simulink model "aaa"  (R2016b)
settings: Solver=ode4  StartTime=0.0  StopTime=inf  FixedStep=0.002  RelTol=1e-3  EnableMultiTasking=on
libraries: slrtlib x3
(part 5 of 5)

== stateflow chart aaa/tiaoshimoshi/jinjichuli7 ==
  state MANUAL
    state kaigai [parallel]
      settings: executionOrder=1
      state A
        entry:kghx=0;
      state on
        entry:kghx=1;
      (default) -> MANUAL.kaigai.A
      MANUAL.kaigai.on -> MANUAL.kaigai.A : [kaigai==0]
      MANUAL.kaigai.A -> MANUAL.kaigai.on : [kaigai==1]
    state guangai [parallel]
      settings: executionOrder=2
      state A
        entry:gghx=0;
      state on
        entry:gghx=1;
      (default) -> MANUAL.guangai.A
      MANUAL.guangai.on -> MANUAL.guangai.A : [guangai==0]
      MANUAL.guangai.A -> MANUAL.guangai.on : [guangai==1]
    state songkai [parallel]
      settings: executionOrder=3
      state A
        entry:skhx=0;
      state on
        entry:skhx=1;
      (default) -> MANUAL.songkai.A
      MANUAL.songkai.on -> MANUAL.songkai.A : [songkai==0]
      MANUAL.songkai.A -> MANUAL.songkai.on : [songkai==1]
    state yajin [parallel]
      settings: executionOrder=4
      state A
        entry:yjhx=0;
      state on
        entry:yjhx=1;
      (default) -> MANUAL.yajin.A
      MANUAL.yajin.on -> MANUAL.yajin.A : [yajin==0]
      MANUAL.yajin.A -> MANUAL.yajin.on : [yajin==1]
    state suoding [parallel]
      settings: executionOrder=5
      state A
        entry:yjhx=0;
      state on
        entry:yjhx=1;
      (default) -> MANUAL.suoding.A
      MANUAL.suoding.on -> MANUAL.suoding.A : [suoding==0]
      MANUAL.suoding.A -> MANUAL.suoding.on : [suoding==1]
    state jiesuo [parallel]
      settings: executionOrder=6
      state A
        entry:skhx=0;
      state on
        entry:skhx=1;
      (default) -> MANUAL.jiesuo.A
      MANUAL.jiesuo.on -> MANUAL.jiesuo.A : [jiesuo==0]
      MANUAL.jiesuo.A -> MANUAL.jiesuo.on : [jiesuo==1]
  state off1
  state on1
    entry:
    skhx=0;
    kghx=0;
    yjhx=0;
    gghx=0;
  state end
    en:
    skhx=0;
    kghx=0;
    yjhx=0;
    gghx=0
  (default) -> off1
  off1 -> on1 : [tiaoshi==1]
  on1 -> MANUAL : after(500,tick)
  MANUAL -> end : [jiting==1]
  data: skhx output double; kghx output double; tiaoshi input double; songkai input; kaigai input; suoding input; jiesuo input; guangai input; yajin input; jiting input; yjhx output double; gghx output double

== stateflow chart aaa/Subsystem1/Chart ==
  state off
    entry:
    kaigaihuanchongyichang=0;
    t=0;
  state on
    entry:
    t=t+0.002;
  state on1
    entry:
    kaigaihuanchongyichang=1;
  (default) -> off
  off -> on : [kaigaihuanxiang==1]
  on -> on [order 1] : [t<=8&&kaigaihuanchong==0]
  on -> on1 [order 2] : [t>8&&kaigaihuanchong==1]
  data: t local; kaigaihuanchongyichang output; kaigaihuanchong input; kaigaihuanxiang input

== stateflow chart aaa/Subsystem1/Chart1 ==
  state off
    entry:
    guangaihuanchongyichang=0;
    t=0;
  state on
    entry:
    t=t+0.002;
  state on1
    entry:
    guangaihuanchongyichang=1;
  (default) -> off
  off -> on : [guangaihuanxiang==1]
  on -> on [order 1] : [t<=8&&guangaihuanchong==0]
  on -> on1 [order 2] : [t>8&&guangaihuanchong==1]
  data: guangaihuanchong input; t local; guangaihuanxiang input; guangaihuanchongyichang output
